simulink model "Simulink_Control_BlueROVtest6"  (R2022b)
settings: Solver=VariableStepAuto  StartTime=0.0  StopTime=20  RelTol=1e-3
model workspace (MAT data in the model file):
  Minv : Simulink.Parameter (value not decoded)
values from neighbouring files (symbols this model uses):
  B = 0    [Control_BlueROV_Modo_Deslizante.m]
  C = 1    [Control_BlueROV_Modo_Deslizante.m]
  epsilong = 1    [Control_BlueROV_Modo_Deslizante.m]
  Ix = 0.1836    [Control_BlueROV_Modo_Deslizante.m]
  Ixy = 0    [Control_BlueROV_Modo_Deslizante.m]
  Ixz = 0    [Control_BlueROV_Modo_Deslizante.m]
  Iy = 0.2181    [Control_BlueROV_Modo_Deslizante.m]
  Iyz = -0.0021    [Control_BlueROV_Modo_Deslizante.m]
  Iz = 0.1482    [Control_BlueROV_Modo_Deslizante.m]
  K = 5    [Control_BlueROV_Modo_Deslizante.m]
  Kp = -5.005    [Control_BlueROV_Modo_Deslizante.m]
  Kpdot = -0.8576    [Control_BlueROV_Modo_Deslizante.m]
  Kpp = -80.25    [Control_BlueROV_Modo_Deslizante.m]
  m = 10.7668    [Control_BlueROV_Modo_Deslizante.m]
  M = Mrb+Ma    [Control_BlueROV_Modo_Deslizante.m]
  Minv = inv(M)    [Control_BlueROV_Modo_Deslizante.m]
  Mq = -5.005    [Control_BlueROV_Modo_Deslizante.m]
  Mqdot = -1.1214    [Control_BlueROV_Modo_Deslizante.m]
  Mqq = -80.25    [Control_BlueROV_Modo_Deslizante.m]
  Nr = -0.004    [Control_BlueROV_Modo_Deslizante.m]
  Nrdot = -0.7399    [Control_BlueROV_Modo_Deslizante.m]
  Nrr = -0.2506    [Control_BlueROV_Modo_Deslizante.m]
  W = 0    [Control_BlueROV_Modo_Deslizante.m]
  xb = 0    [Control_BlueROV_Modo_Deslizante.m]
  xg = 0    [Control_BlueROV_Modo_Deslizante.m]
  Xu = -0.0048    [Control_BlueROV_Modo_Deslizante.m]
  Xudot = -4.9063    [Control_BlueROV_Modo_Deslizante.m]
  Xuu = -30.61    [Control_BlueROV_Modo_Deslizante.m]
  yb = 0    [Control_BlueROV_Modo_Deslizante.m]
  yg = 0    [Control_BlueROV_Modo_Deslizante.m]
  Yv = -0.2437    [Control_BlueROV_Modo_Deslizante.m]
  Yvdot = -9.9210    (= -9.921)    [Control_BlueROV_Modo_Deslizante.m]
  Yvv = -38.0036    [Control_BlueROV_Modo_Deslizante.m]
  zb = 0.02    [Control_BlueROV_Modo_Deslizante.m]
  zg = 0    [Control_BlueROV_Modo_Deslizante.m]
  Zw = -0.0094    [Control_BlueROV_Modo_Deslizante.m]
  Zwdot = -17.6159    [Control_BlueROV_Modo_Deslizante.m]
  Zww = -62.5364    [Control_BlueROV_Modo_Deslizante.m]
libraries: simulink x1
(part 2 of 3)

== system Simulink_Control_BlueROVtest6/BlueRov2Heavy/C(v)/Subsystem13 ==
  In1 : Inport
  In2 : Inport  Port=2
  In3 : Inport  Port=3
  In4 : Inport  Port=4
  Add4 : Sum  Inputs=+++
  Add8 : Sum
  Constant : Constant  Value=Iyz
  Constant1 : Constant  Value=-Iy
  Constant10 : Constant  Value=Ixy
  Constant11 : Constant  Value=Mqdot
  Product{1,19..21} (4 alike) : Product
  Out1 : Outport  VectorParamsAs1DForOutWhenUnconnected=off
  wires:
  In3/1 -> Product1/2
  In4/1 -> Product21/2
  Constant1/1 -> Product1/1
  Product1/1 -> Add4/3
  Product20/1 -> Add4/2
  Constant11/1 -> Product21/1
  Add4/1 -> Add8/1
  Product19/1 -> Add4/1
  Constant/1 -> Product19/1
  Product21/1 -> Add8/2
  Constant10/1 -> Product20/1
  Add8/1 -> Out1/1
  In1/1 -> Product19/2
  In2/1 -> Product20/2

== system Simulink_Control_BlueROVtest6/BlueRov2Heavy/C(v)/Subsystem14 ==
  In1 : Inport
  In2 : Inport  Port=2
  In3 : Inport  Port=3
  Add4 : Sum  Inputs=+-
  Add8 : Sum
  Constant : Constant  Value=xg
  Constant10 : Constant
  Constant11 : Constant  Value=Zwdot
  Gain : Gain  Gain=m
  Product19 : Product
  Product20 : Product
  Product21 : Product
  Out1 : Outport  VectorParamsAs1DForOutWhenUnconnected=off
  wires:
  Product20/1 -> Add4/2
  Constant11/1 -> Product21/1
  Gain/1 -> Add8/1
  Product19/1 -> Add4/1
  Constant/1 -> Product19/1
  Product21/1 -> Add8/2
  Add4/1 -> Gain/1
  Constant10/1 -> Product20/1
  Add8/1 -> Out1/1
  In1/1 -> Product19/2
  In3/1 -> Product21/2
  In2/1 -> Product20/2

== system Simulink_Control_BlueROVtest6/BlueRov2Heavy/C(v)/Subsystem15 ==
  In1 : Inport
  In2 : Inport  Port=2
  In3 : Inport  Port=3
  Add4 : Sum
  Add8 : Sum
  Constant : Constant  Value=zg
  Constant10 : Constant
  Constant11 : Constant  Value=-Xudot
  Gain : Gain  Gain=m
  Product19 : Product
  Product20 : Product
  Product21 : Product
  Out1 : Outport  VectorParamsAs1DForOutWhenUnconnected=off
  wires:
  In2/1 -> Product20/2
  In3/1 -> Product21/2
  In1/1 -> Product19/2
  Add8/1 -> Out1/1
  Constant10/1 -> Product20/1
  Add4/1 -> Gain/1
  Product21/1 -> Add8/2
  Constant/1 -> Product19/1
  Product19/1 -> Add4/1
  Gain/1 -> Add8/1
  Constant11/1 -> Product21/1
  Product20/1 -> Add4/2

== system Simulink_Control_BlueROVtest6/BlueRov2Heavy/C(v)/Subsystem16 ==
  In1 : Inport
  In2 : Inport  Port=2
  Add4 : Sum
  Constant : Constant  Value=zg
  Constant10 : Constant  Value=xg
  Gain : Gain  Gain=-m
  Product19 : Product
  Product20 : Product
  Out1 : Outport  VectorParamsAs1DForOutWhenUnconnected=off
  wires:
  Product20/1 -> Add4/2
  Product19/1 -> Add4/1
  In1/1 -> Product19/2
  Constant/1 -> Product19/1
  Gain/1 -> Out1/1
  Constant10/1 -> Product20/1
  Add4/1 -> Gain/1
  In2/1 -> Product20/2

== system Simulink_Control_BlueROVtest6/BlueRov2Heavy/C(v)/Subsystem17 ==
  In1 : Inport
  In2 : Inport  Port=2
  In3 : Inport  Port=3
  In4 : Inport  Port=4
  Add4 : Sum  Inputs=+++
  Add8 : Sum
  Constant : Constant  Value=Iyz
  Constant1 : Constant  Value=-Iz
  Constant10 : Constant  Value=Ixz
  Constant11 : Constant  Value=Nrdot
  Product{1,19..21} (4 alike) : Product
  Out1 : Outport  VectorParamsAs1DForOutWhenUnconnected=off
  wires:
  In3/1 -> Product1/2
  In4/1 -> Product21/2
  Constant1/1 -> Product1/1
  Product1/1 -> Add4/3
  Product20/1 -> Add4/2
  Constant11/1 -> Product21/1
  Add4/1 -> Add8/1
  Product19/1 -> Add4/1
  Constant/1 -> Product19/1
  Product21/1 -> Add8/2
  Constant10/1 -> Product20/1
  Add8/1 -> Out1/1
  In1/1 -> Product19/2
  In2/1 -> Product20/2

== system Simulink_Control_BlueROVtest6/BlueRov2Heavy/C(v)/Subsystem18 ==
  In1 : Inport
  In2 : Inport  Port=2
  In3 : Inport  Port=3
  In4 : Inport  Port=4
  Add4 : Sum  Inputs=+++
  Add8 : Sum
  Constant : Constant  Value=-Ixz
  Constant1 : Constant  Value=Ix
  Constant10 : Constant  Value=-Ixy
  Constant11 : Constant  Value=-Kpdot
  Product{1,19..21} (4 alike) : Product
  Out1 : Outport  VectorParamsAs1DForOutWhenUnconnected=off
  wires:
  In2/1 -> Product20/2
  In1/1 -> Product19/2
  Add8/1 -> Out1/1
  Constant10/1 -> Product20/1
  Product21/1 -> Add8/2
  Constant/1 -> Product19/1
  Product19/1 -> Add4/1
  Add4/1 -> Add8/1
  Constant11/1 -> Product21/1
  Product20/1 -> Add4/2
  Product1/1 -> Add4/3
  Constant1/1 -> Product1/1
  In4/1 -> Product21/2
  In3/1 -> Product1/2

== system Simulink_Control_BlueROVtest6/BlueRov2Heavy/C(v)/Subsystem19 ==
  In1 : Inport
  In2 : Inport  Port=2
  In3 : Inport  Port=3
  Add4 : Sum
  Add8 : Sum
  Constant : Constant  Value=xg
  Constant10 : Constant
  Constant11 : Constant  Value=-Yvdot
  Gain : Gain  Gain=m
  Product19 : Product
  Product20 : Product
  Product21 : Product
  Out1 : Outport  VectorParamsAs1DForOutWhenUnconnected=off
  wires:
  In2/1 -> Product20/2
  In3/1 -> Product21/2
  In1/1 -> Product19/2
  Add8/1 -> Out1/1
  Constant10/1 -> Product20/1
  Add4/1 -> Gain/1
  Product21/1 -> Add8/2
  Constant/1 -> Product19/1
  Product19/1 -> Add4/1
  Gain/1 -> Add8/1
  Constant11/1 -> Product21/1
  Product20/1 -> Add4/2

== system Simulink_Control_BlueROVtest6/BlueRov2Heavy/C(v)/Subsystem2 ==
  In1 : Inport
  In2 : Inport  Port=2
  In3 : Inport  Port=3
  Add10 : Sum  Inputs=-+
  Add9 : Sum
  Constant12 : Constant  Value=xg
  Constant13 : Constant
  Constant14 : Constant  Value=Yvdot
  Gain1 : Gain  Gain=m
  Product22 : Product
  Product23 : Product
  Product24 : Product
  Out1 : Outport  VectorParamsAs1DForOutWhenUnconnected=off
  wires:
  In1/1 -> Product22/2
  Constant14/1 -> Product24/1
  Add9/1 -> Gain1/1
  Constant12/1 -> Product22/1
  Product23/1 -> Add9/2
  Gain1/1 -> Add10/1
  Constant13/1 -> Product23/1
  Product24/1 -> Add10/2
  Product22/1 -> Add9/1
  In3/1 -> Product24/2
  Add10/1 -> Out1/1
  In2/1 -> Product23/2

== system Simulink_Control_BlueROVtest6/BlueRov2Heavy/C(v)/Subsystem20 ==
  In1 : Inport
  In2 : Inport  Port=2
  In3 : Inport  Port=3
  Add4 : Sum
  Add8 : Sum
  Constant : Constant  Value=yg
  Constant10 : Constant  Value=-1
  Constant11 : Constant  Value=Xudot
  Gain : Gain  Gain=m
  Product19 : Product
  Product20 : Product
  Product21 : Product
  Out1 : Outport  VectorParamsAs1DForOutWhenUnconnected=off
  wires:
  Product20/1 -> Add4/2
  Constant11/1 -> Product21/1
  Gain/1 -> Add8/1
  Product19/1 -> Add4/1
  Constant/1 -> Product19/1
  Product21/1 -> Add8/2
  Add4/1 -> Gain/1
  Constant10/1 -> Product20/1
  Add8/1 -> Out1/1
  In1/1 -> Product19/2
  In3/1 -> Product21/2
  In2/1 -> Product20/2

== system Simulink_Control_BlueROVtest6/BlueRov2Heavy/C(v)/Subsystem21 ==
  In1 : Inport
  In2 : Inport  Port=2
  Add4 : Sum
  Constant : Constant  Value=xg
  Constant10 : Constant  Value=yg
  Gain : Gain  Gain=-m
  Product19 : Product
  Product20 : Product
  Out1 : Outport  VectorParamsAs1DForOutWhenUnconnected=off
  wires:
  In2/1 -> Product20/2
  Add4/1 -> Gain/1
  Constant10/1 -> Product20/1
  Gain/1 -> Out1/1
  Constant/1 -> Product19/1
  In1/1 -> Product19/2
  Product19/1 -> Add4/1
  Product20/1 -> Add4/2

== system Simulink_Control_BlueROVtest6/BlueRov2Heavy/C(v)/Subsystem22 ==
  In1 : Inport
  In2 : Inport  Port=2
  In3 : Inport  Port=3
  In4 : Inport  Port=4
  Add4 : Sum  Inputs=+++
  Add8 : Sum
  Constant : Constant  Value=-Iyz
  Constant1 : Constant  Value=Iy
  Constant10 : Constant  Value=-Ixy
  Constant11 : Constant  Value=-Mqdot
  Product{1,19..21} (4 alike) : Product
  Out1 : Outport  VectorParamsAs1DForOutWhenUnconnected=off
  wires:
  In2/1 -> Product20/2
  In1/1 -> Product19/2
  Add8/1 -> Out1/1
  Constant10/1 -> Product20/1
  Product21/1 -> Add8/2
  Constant/1 -> Product19/1
  Product19/1 -> Add4/1
  Add4/1 -> Add8/1
  Constant11/1 -> Product21/1
  Product20/1 -> Add4/2
  Product1/1 -> Add4/3
  Constant1/1 -> Product1/1
  In4/1 -> Product21/2
  In3/1 -> Product1/2

== system Simulink_Control_BlueROVtest6/BlueRov2Heavy/C(v)/Subsystem23 ==
  In1 : Inport
  In2 : Inport  Port=2
  In3 : Inport  Port=3
  In4 : Inport  Port=4
  Add4 : Sum  Inputs=+++
  Add8 : Sum
  Constant : Constant  Value=Ixz
  Constant1 : Constant  Value=-Ix
  Constant10 : Constant  Value=Ixy
  Constant11 : Constant  Value=Kpdot
  Product{1,19..21} (4 alike) : Product
  Out1 : Outport  VectorParamsAs1DForOutWhenUnconnected=off
  wires:
  In3/1 -> Product1/2
  In4/1 -> Product21/2
  Constant1/1 -> Product1/1
  Product1/1 -> Add4/3
  Product20/1 -> Add4/2
  Constant11/1 -> Product21/1
  Add4/1 -> Add8/1
  Product19/1 -> Add4/1
  Constant/1 -> Product19/1
  Product21/1 -> Add8/2
  Constant10/1 -> Product20/1
  Add8/1 -> Out1/1
  In1/1 -> Product19/2
  In2/1 -> Product20/2

== system Simulink_Control_BlueROVtest6/BlueRov2Heavy/C(v)/Subsystem3 ==
  In1 : Inport
  In2 : Inport  Port=2
  In3 : Inport  Port=3
  Add4 : Sum
  Add8 : Sum  Inputs=-+
  Constant : Constant  Value=yg
  Constant10 : Constant
  Constant11 : Constant  Value=Zwdot
  Gain : Gain  Gain=m
  Product19 : Product
  Product20 : Product
  Product21 : Product
  Out1 : Outport  VectorParamsAs1DForOutWhenUnconnected=off
  wires:
  In2/1 -> Product20/2
  In3/1 -> Product21/2
  In1/1 -> Product19/2
  Add8/1 -> Out1/1
  Constant10/1 -> Product20/1
  Add4/1 -> Gain/1
  Product21/1 -> Add8/2
  Constant/1 -> Product19/1
  Product19/1 -> Add4/1
  Gain/1 -> Add8/1
  Constant11/1 -> Product21/1
  Product20/1 -> Add4/2

== system Simulink_Control_BlueROVtest6/BlueRov2Heavy/C(v)/Subsystem4 ==
  In1 : Inport
  In2 : Inport  Port=2
  Add4 : Sum
  Constant : Constant  Value=zg
  Constant10 : Constant  Value=xg
  Gain : Gain  Gain=m
  Product19 : Product
  Product20 : Product
  Out1 : Outport  VectorParamsAs1DForOutWhenUnconnected=off
  wires:
  In2/1 -> Product20/2
  Add4/1 -> Gain/1
  Constant10/1 -> Product20/1
  Gain/1 -> Out1/1
  Constant/1 -> Product19/1
  In1/1 -> Product19/2
  Product19/1 -> Add4/1
  Product20/1 -> Add4/2

== system Simulink_Control_BlueROVtest6/BlueRov2Heavy/C(v)/Subsystem5 ==
  In1 : Inport
  In2 : Inport  Port=2
  In3 : Inport  Port=3
  Add4 : Sum  Inputs=+-
  Add8 : Sum  Inputs=-+
  Constant : Constant  Value=yg
  Constant10 : Constant
  Constant11 : Constant  Value=-Xudot
  Gain : Gain  Gain=m
  Product19 : Product
  Product20 : Product
  Product21 : Product
  Out1 : Outport  VectorParamsAs1DForOutWhenUnconnected=off
  wires:
  Product20/1 -> Add4/2
  Constant11/1 -> Product21/1
  Gain/1 -> Add8/1
  Product19/1 -> Add4/1
  Constant/1 -> Product19/1
  Product21/1 -> Add8/2
  Add4/1 -> Gain/1
  Constant10/1 -> Product20/1
  Add8/1 -> Out1/1
  In1/1 -> Product19/2
  In3/1 -> Product21/2
  In2/1 -> Product20/2

== system Simulink_Control_BlueROVtest6/BlueRov2Heavy/C(v)/Subsystem6 ==
  In1 : Inport
  In2 : Inport  Port=2
  In3 : Inport  Port=3
  Add4 : Sum  Inputs=+-
  Add8 : Sum  Inputs=-+
  Constant : Constant  Value=zg
  Constant10 : Constant
  Constant11 : Constant  Value=-Yvdot
  Gain : Gain  Gain=m
  Product19 : Product
  Product20 : Product
  Product21 : Product
  Out1 : Outport  VectorParamsAs1DForOutWhenUnconnected=off
  wires:
  In2/1 -> Product20/2
  In3/1 -> Product21/2
  In1/1 -> Product19/2
  Add8/1 -> Out1/1
  Constant10/1 -> Product20/1
  Add4/1 -> Gain/1
  Product21/1 -> Add8/2
  Constant/1 -> Product19/1
  Product19/1 -> Add4/1
  Gain/1 -> Add8/1
  Constant11/1 -> Product21/1
  Product20/1 -> Add4/2

== system Simulink_Control_BlueROVtest6/BlueRov2Heavy/C(v)/Subsystem7 ==
  In1 : Inport
  In2 : Inport  Port=2
  In3 : Inport  Port=3
  Add4 : Sum
  Add8 : Sum  Inputs=-+
  Constant : Constant  Value=zg
  Constant10 : Constant
  Constant11 : Constant  Value=Xudot
  Gain : Gain  Gain=m
  Product19 : Product
  Product20 : Product
  Product21 : Product
  Out1 : Outport  VectorParamsAs1DForOutWhenUnconnected=off
  wires:
  Product20/1 -> Add4/2
  Constant11/1 -> Product21/1
  Gain/1 -> Add8/1
  Product19/1 -> Add4/1
  Constant/1 -> Product19/1
  Product21/1 -> Add8/2
  Add4/1 -> Gain/1
  Constant10/1 -> Product20/1
  Add8/1 -> Out1/1
  In1/1 -> Product19/2
  In3/1 -> Product21/2
  In2/1 -> Product20/2

== system Simulink_Control_BlueROVtest6/BlueRov2Heavy/C(v)/Subsystem8 ==
  In1 : Inport
  In2 : Inport  Port=2
  Add4 : Sum
  Constant : Constant  Value=xg
  Constant10 : Constant  Value=yg
  Gain : Gain  Gain=m
  Product19 : Product
  Product20 : Product
  Out1 : Outport  VectorParamsAs1DForOutWhenUnconnected=off
  wires:
  In2/1 -> Product20/2
  Add4/1 -> Gain/1
  Constant10/1 -> Product20/1
  Gain/1 -> Out1/1
  Constant/1 -> Product19/1
  In1/1 -> Product19/2
  Product19/1 -> Add4/1
  Product20/1 -> Add4/2

== system Simulink_Control_BlueROVtest6/BlueRov2Heavy/C(v)/Subsystem9 ==
  In1 : Inport
  In2 : Inport  Port=2
  Add4 : Sum
  Constant : Constant  Value=yg
  Constant10 : Constant  Value=zg
  Gain : Gain  Gain=-m
  Product19 : Product
  Product20 : Product
  Out1 : Outport  VectorParamsAs1DForOutWhenUnconnected=off
  wires:
  In2/1 -> Product20/2
  Add4/1 -> Gain/1
  Constant10/1 -> Product20/1
  Gain/1 -> Out1/1
  Constant/1 -> Product19/1
  In1/1 -> Product19/2
  Product19/1 -> Add4/1
  Product20/1 -> Add4/2

== system Simulink_Control_BlueROVtest6/BlueRov2Heavy/J(n)/Subsystem1 ==
  In1 : Inport
  In2 : Inport  Port=2
  Product6 : Product
  Out1 : Outport  VectorParamsAs1DForOutWhenUnconnected=off
  wires:
  In1/1 -> Product6/1
  In2/1 -> Product6/2
  Product6/1 -> Out1/1

== system Simulink_Control_BlueROVtest6/BlueRov2Heavy/J(n)/Subsystem10 ==
  In1 : Inport
  In2 : Inport  Port=2
  Product6 : Product
  Out1 : Outport  VectorParamsAs1DForOutWhenUnconnected=off
  wires:
  In1/1 -> Product6/1
  In2/1 -> Product6/2
  Product6/1 -> Out1/1

== system Simulink_Control_BlueROVtest6/BlueRov2Heavy/J(n)/Subsystem11 ==
  In1 : Inport
  In2 : Inport  Port=2
  Product6 : Product
  Out1 : Outport  VectorParamsAs1DForOutWhenUnconnected=off
  wires:
  In1/1 -> Product6/1
  In2/1 -> Product6/2
  Product6/1 -> Out1/1

== system Simulink_Control_BlueROVtest6/BlueRov2Heavy/J(n)/Subsystem12 ==
  In1 : Inport
  In2 : Inport  Port=2
  Product6 : Product
  Out1 : Outport  VectorParamsAs1DForOutWhenUnconnected=off
  wires:
  In1/1 -> Product6/1
  In2/1 -> Product6/2
  Product6/1 -> Out1/1

== system Simulink_Control_BlueROVtest6/BlueRov2Heavy/J(n)/Subsystem2 ==
  In1 : Inport
  In2 : Inport  Port=2
  In3 : Inport  Port=3
  In4 : Inport  Port=4
  In5 : Inport  Port=5
  Add7 : Sum
  Product37 : Product
  Product38 : Product  Inputs=3
  Out1 : Outport  VectorParamsAs1DForOutWhenUnconnected=off
  wires:
  In5/1 -> Product38/3
  In4/1 -> Product38/2
  In3/1 -> Product38/1
  In2/1 -> Product37/2
  In1/1 -> Product37/1
  Product37/1 -> Add7/1
  Add7/1 -> Out1/1
  Product38/1 -> Add7/2

== system Simulink_Control_BlueROVtest6/BlueRov2Heavy/J(n)/Subsystem3 ==
  In1 : Inport
  In2 : Inport  Port=2
  Product6 : Product
  Out1 : Outport  VectorParamsAs1DForOutWhenUnconnected=off
  wires:
  Product6/1 -> Out1/1
  In2/1 -> Product6/2
  In1/1 -> Product6/1

== system Simulink_Control_BlueROVtest6/BlueRov2Heavy/J(n)/Subsystem4 ==
  In1 : Inport
  In2 : Inport  Port=2
  In3 : Inport  Port=3
  In4 : Inport  Port=4
  In5 : Inport  Port=5
  Add7 : Sum  Inputs=-+
  Product37 : Product
  Product38 : Product  Inputs=3
  Out1 : Outport  VectorParamsAs1DForOutWhenUnconnected=off
  wires:
  Product38/1 -> Add7/2
  Add7/1 -> Out1/1
  Product37/1 -> Add7/1
  In1/1 -> Product37/1
  In2/1 -> Product37/2
  In3/1 -> Product38/1
  In4/1 -> Product38/2
  In5/1 -> Product38/3

== system Simulink_Control_BlueROVtest6/BlueRov2Heavy/J(n)/Subsystem5 ==
  In1 : Inport
  In2 : Inport  Port=2
  In3 : Inport  Port=3
  In4 : Inport  Port=4
  In5 : Inport  Port=5
  Add7 : Sum
  Product37 : Product
  Product38 : Product  Inputs=3
  Out1 : Outport  VectorParamsAs1DForOutWhenUnconnected=off
  wires:
  Product38/1 -> Add7/2
  Add7/1 -> Out1/1
  Product37/1 -> Add7/1
  In1/1 -> Product37/1
  In2/1 -> Product37/2
  In3/1 -> Product38/1
  In4/1 -> Product38/2
  In5/1 -> Product38/3

== system Simulink_Control_BlueROVtest6/BlueRov2Heavy/J(n)/Subsystem6 ==
  In1 : Inport
  In2 : Inport  Port=2
  In3 : Inport  Port=3
  In4 : Inport  Port=4
  In5 : Inport  Port=5
  Add7 : Sum  Inputs=-+
  Product37 : Product
  Product38 : Product  Inputs=3
  Out1 : Outport  VectorParamsAs1DForOutWhenUnconnected=off
  wires:
  In5/1 -> Product38/3
  In4/1 -> Product38/2
  In3/1 -> Product38/1
  In2/1 -> Product37/2
  In1/1 -> Product37/1
  Product37/1 -> Add7/1
  Add7/1 -> Out1/1
  Product38/1 -> Add7/2

== system Simulink_Control_BlueROVtest6/BlueRov2Heavy/J(n)/Subsystem7 ==
  In1 : Inport
  In2 : Inport  Port=2
  Product6 : Product
  Out1 : Outport  VectorParamsAs1DForOutWhenUnconnected=off
  wires:
  In1/1 -> Product6/1
  In2/1 -> Product6/2
  Product6/1 -> Out1/1

== system Simulink_Control_BlueROVtest6/BlueRov2Heavy/J(n)/Subsystem8 ==
  In1 : Inport
  In2 : Inport  Port=2
  Product6 : Product
  Out1 : Outport  VectorParamsAs1DForOutWhenUnconnected=off
  wires:
  Product6/1 -> Out1/1
  In2/1 -> Product6/2
  In1/1 -> Product6/1

== system Simulink_Control_BlueROVtest6/BlueRov2Heavy/J(n)/Subsystem9 ==
  In1 : Inport
  In2 : Inport  Port=2
  Product6 : Product
  Out1 : Outport  VectorParamsAs1DForOutWhenUnconnected=off
  wires:
  In1/1 -> Product6/1
  In2/1 -> Product6/2
  Product6/1 -> Out1/1

== system Simulink_Control_BlueROVtest6/FeedBackData1/J(n)/Subsystem1 ==
  In1 : Inport
  In2 : Inport  Port=2
  Product6 : Product
  Out1 : Outport  VectorParamsAs1DForOutWhenUnconnected=off
  wires:
  In1/1 -> Product6/1
  In2/1 -> Product6/2
  Product6/1 -> Out1/1

== system Simulink_Control_BlueROVtest6/FeedBackData1/J(n)/Subsystem10 ==
  In1 : Inport
  In2 : Inport  Port=2
  Product6 : Product
  Out1 : Outport  VectorParamsAs1DForOutWhenUnconnected=off
  wires:
  In1/1 -> Product6/1
  In2/1 -> Product6/2
  Product6/1 -> Out1/1

== system Simulink_Control_BlueROVtest6/FeedBackData1/J(n)/Subsystem11 ==
  In1 : Inport
  In2 : Inport  Port=2
  Product6 : Product
  Out1 : Outport  VectorParamsAs1DForOutWhenUnconnected=off
  wires:
  In1/1 -> Product6/1
  In2/1 -> Product6/2
  Product6/1 -> Out1/1

== system Simulink_Control_BlueROVtest6/FeedBackData1/J(n)/Subsystem12 ==
  In1 : Inport
  In2 : Inport  Port=2
  Product6 : Product
  Out1 : Outport  VectorParamsAs1DForOutWhenUnconnected=off
  wires:
  In1/1 -> Product6/1
  In2/1 -> Product6/2
  Product6/1 -> Out1/1

== system Simulink_Control_BlueROVtest6/FeedBackData1/J(n)/Subsystem2 ==
  In1 : Inport
  In2 : Inport  Port=2
  In3 : Inport  Port=3
  In4 : Inport  Port=4
  In5 : Inport  Port=5
  Add7 : Sum
  Product37 : Product
  Product38 : Product  Inputs=3
  Out1 : Outport  VectorParamsAs1DForOutWhenUnconnected=off
  wires:
  In5/1 -> Product38/3
  In4/1 -> Product38/2
  In3/1 -> Product38/1
  In2/1 -> Product37/2
  In1/1 -> Product37/1
  Product37/1 -> Add7/1
  Add7/1 -> Out1/1
  Product38/1 -> Add7/2

== system Simulink_Control_BlueROVtest6/FeedBackData1/J(n)/Subsystem3 ==
  In1 : Inport
  In2 : Inport  Port=2
  Product6 : Product
  Out1 : Outport  VectorParamsAs1DForOutWhenUnconnected=off
  wires:
  Product6/1 -> Out1/1
  In2/1 -> Product6/2
  In1/1 -> Product6/1

== system Simulink_Control_BlueROVtest6/FeedBackData1/J(n)/Subsystem4 ==
  In1 : Inport
  In2 : Inport  Port=2
  In3 : Inport  Port=3
  In4 : Inport  Port=4
  In5 : Inport  Port=5
  Add7 : Sum  Inputs=-+
  Product37 : Product
  Product38 : Product  Inputs=3
  Out1 : Outport  VectorParamsAs1DForOutWhenUnconnected=off
  wires:
  Product38/1 -> Add7/2
  Add7/1 -> Out1/1
  Product37/1 -> Add7/1
  In1/1 -> Product37/1
  In2/1 -> Product37/2
  In3/1 -> Product38/1
  In4/1 -> Product38/2
  In5/1 -> Product38/3

== system Simulink_Control_BlueROVtest6/FeedBackData1/J(n)/Subsystem5 ==
  In1 : Inport
  In2 : Inport  Port=2
  In3 : Inport  Port=3
  In4 : Inport  Port=4
  In5 : Inport  Port=5
  Add7 : Sum
  Product37 : Product
  Product38 : Product  Inputs=3
  Out1 : Outport  VectorParamsAs1DForOutWhenUnconnected=off
  wires:
  Product38/1 -> Add7/2
  Add7/1 -> Out1/1
  Product37/1 -> Add7/1
  In1/1 -> Product37/1
  In2/1 -> Product37/2
  In3/1 -> Product38/1
  In4/1 -> Product38/2
  In5/1 -> Product38/3

== system Simulink_Control_BlueROVtest6/FeedBackData1/J(n)/Subsystem6 ==
  In1 : Inport
  In2 : Inport  Port=2
  In3 : Inport  Port=3
  In4 : Inport  Port=4
  In5 : Inport  Port=5
  Add7 : Sum  Inputs=-+
  Product37 : Product
  Product38 : Product  Inputs=3
  Out1 : Outport  VectorParamsAs1DForOutWhenUnconnected=off
  wires:
  In5/1 -> Product38/3
  In4/1 -> Product38/2
  In3/1 -> Product38/1
  In2/1 -> Product37/2
  In1/1 -> Product37/1
  Product37/1 -> Add7/1
  Add7/1 -> Out1/1
  Product38/1 -> Add7/2

== system Simulink_Control_BlueROVtest6/FeedBackData1/J(n)/Subsystem7 ==
  In1 : Inport
  In2 : Inport  Port=2
  Product6 : Product
  Out1 : Outport  VectorParamsAs1DForOutWhenUnconnected=off
  wires:
  In1/1 -> Product6/1
  In2/1 -> Product6/2
  Product6/1 -> Out1/1

== system Simulink_Control_BlueROVtest6/FeedBackData1/J(n)/Subsystem8 ==
  In1 : Inport
  In2 : Inport  Port=2
  Product6 : Product
  Out1 : Outport  VectorParamsAs1DForOutWhenUnconnected=off
  wires:
  Product6/1 -> Out1/1
  In2/1 -> Product6/2
  In1/1 -> Product6/1

== system Simulink_Control_BlueROVtest6/FeedBackData1/J(n)/Subsystem9 ==
  In1 : Inport
  In2 : Inport  Port=2
  Product6 : Product
  Out1 : Outport  VectorParamsAs1DForOutWhenUnconnected=off
  wires:
  In1/1 -> Product6/1
  In2/1 -> Product6/2
  Product6/1 -> Out1/1

== system Simulink_Control_BlueROVtest6/Sliding Mode Control/C(v)/Subsystem ==
  In1 : Inport
  In2 : Inport  Port=2
  Add4 : Sum
  Constant : Constant  Value=zg
  Constant10 : Constant  Value=yg
  Gain : Gain  Gain=m
  Product19 : Product
  Product20 : Product
  Out1 : Outport  VectorParamsAs1DForOutWhenUnconnected=off
  wires:
  Product20/1 -> Add4/2
  Product19/1 -> Add4/1
  In1/1 -> Product19/2
  Constant/1 -> Product19/1
  Gain/1 -> Out1/1
  Constant10/1 -> Product20/1
  Add4/1 -> Gain/1
  In2/1 -> Product20/2

== system Simulink_Control_BlueROVtest6/Sliding Mode Control/C(v)/Subsystem1 ==
  In1 : Inport
  In2 : Inport  Port=2
  In3 : Inport  Port=3
  Add4 : Sum  Inputs=+-
  Add8 : Sum  Inputs=-+
  Constant : Constant  Value=xg
  Constant10 : Constant
  Constant11 : Constant  Value=-Zwdot
  Gain : Gain  Gain=m
  Product19 : Product
  Product20 : Product
  Product21 : Product
  Out1 : Outport  VectorParamsAs1DForOutWhenUnconnected=off
  wires:
  Product20/1 -> Add4/2
  Constant11/1 -> Product21/1
  Gain/1 -> Add8/1
  Product19/1 -> Add4/1
  Constant/1 -> Product19/1
  Product21/1 -> Add8/2
  Add4/1 -> Gain/1
  Constant10/1 -> Product20/1
  Add8/1 -> Out1/1
  In1/1 -> Product19/2
  In3/1 -> Product21/2
  In2/1 -> Product20/2

== system Simulink_Control_BlueROVtest6/Sliding Mode Control/C(v)/Subsystem10 ==
  In1 : Inport
  In2 : Inport  Port=2
  In3 : Inport  Port=3
  Add4 : Sum
  Add8 : Sum
  Constant : Constant  Value=yg
  Constant10 : Constant
  Constant11 : Constant  Value=-Zwdot
  Gain : Gain  Gain=m
  Product19 : Product
  Product20 : Product
  Product21 : Product
  Out1 : Outport  VectorParamsAs1DForOutWhenUnconnected=off
  wires:
  In2/1 -> Product20/2
  In3/1 -> Product21/2
  In1/1 -> Product19/2
  Add8/1 -> Out1/1
  Constant10/1 -> Product20/1
  Add4/1 -> Gain/1
  Product21/1 -> Add8/2
  Constant/1 -> Product19/1
  Product19/1 -> Add4/1
  Gain/1 -> Add8/1
  Constant11/1 -> Product21/1
  Product20/1 -> Add4/2

== system Simulink_Control_BlueROVtest6/Sliding Mode Control/C(v)/Subsystem11 ==
  In1 : Inport
  In2 : Inport  Port=2
  In3 : Inport  Port=3
  Add4 : Sum  Inputs=+-
  Add8 : Sum
  Constant : Constant  Value=zg
  Constant10 : Constant
  Constant11 : Constant  Value=Yvdot
  Gain : Gain  Gain=m
  Product19 : Product
  Product20 : Product
  Product21 : Product
  Out1 : Outport  VectorParamsAs1DForOutWhenUnconnected=off
  wires:
  Product20/1 -> Add4/2
  Constant11/1 -> Product21/1
  Gain/1 -> Add8/1
  Product19/1 -> Add4/1
  Constant/1 -> Product19/1
  Product21/1 -> Add8/2
  Add4/1 -> Gain/1
  Constant10/1 -> Product20/1
  Add8/1 -> Out1/1
  In1/1 -> Product19/2
  In3/1 -> Product21/2
  In2/1 -> Product20/2

== system Simulink_Control_BlueROVtest6/Sliding Mode Control/C(v)/Subsystem12 ==
  In1 : Inport
  In2 : Inport  Port=2
  In3 : Inport  Port=3
  In4 : Inport  Port=4
  Add4 : Sum  Inputs=+++
  Add8 : Sum
  Constant : Constant  Value=-Iyz
  Constant1 : Constant  Value=Iz
  Constant10 : Constant  Value=-Ixz
  Constant11 : Constant  Value=-Nrdot
  Product{1,19..21} (4 alike) : Product
  Out1 : Outport  VectorParamsAs1DForOutWhenUnconnected=off
  wires:
  In2/1 -> Product20/2
  In1/1 -> Product19/2
  Add8/1 -> Out1/1
  Constant10/1 -> Product20/1
  Product21/1 -> Add8/2
  Constant/1 -> Product19/1
  Product19/1 -> Add4/1
  Add4/1 -> Add8/1
  Constant11/1 -> Product21/1
  Product20/1 -> Add4/2
  Product1/1 -> Add4/3
  Constant1/1 -> Product1/1
  In4/1 -> Product21/2
  In3/1 -> Product1/2

== system Simulink_Control_BlueROVtest6/Sliding Mode Control/C(v)/Subsystem13 ==
  In1 : Inport
  In2 : Inport  Port=2
  In3 : Inport  Port=3
  In4 : Inport  Port=4
  Add4 : Sum  Inputs=+++
  Add8 : Sum
  Constant : Constant  Value=Iyz
  Constant1 : Constant  Value=-Iy
  Constant10 : Constant  Value=Ixy
  Constant11 : Constant  Value=Mqdot
  Product{1,19..21} (4 alike) : Product
  Out1 : Outport  VectorParamsAs1DForOutWhenUnconnected=off
  wires:
  In3/1 -> Product1/2
  In4/1 -> Product21/2
  Constant1/1 -> Product1/1
  Product1/1 -> Add4/3
  Product20/1 -> Add4/2
  Constant11/1 -> Product21/1
  Add4/1 -> Add8/1
  Product19/1 -> Add4/1
  Constant/1 -> Product19/1
  Product21/1 -> Add8/2
  Constant10/1 -> Product20/1
  Add8/1 -> Out1/1
  In1/1 -> Product19/2
  In2/1 -> Product20/2

== system Simulink_Control_BlueROVtest6/Sliding Mode Control/C(v)/Subsystem14 ==
  In1 : Inport
  In2 : Inport  Port=2
  In3 : Inport  Port=3
  Add4 : Sum  Inputs=+-
  Add8 : Sum
  Constant : Constant  Value=xg
  Constant10 : Constant
  Constant11 : Constant  Value=Zwdot
  Gain : Gain  Gain=m
  Product19 : Product
  Product20 : Product
  Product21 : Product
  Out1 : Outport  VectorParamsAs1DForOutWhenUnconnected=off
  wires:
  Product20/1 -> Add4/2
  Constant11/1 -> Product21/1
  Gain/1 -> Add8/1
  Product19/1 -> Add4/1
  Constant/1 -> Product19/1
  Product21/1 -> Add8/2
  Add4/1 -> Gain/1
  Constant10/1 -> Product20/1
  Add8/1 -> Out1/1
  In1/1 -> Product19/2
  In3/1 -> Product21/2
  In2/1 -> Product20/2

== system Simulink_Control_BlueROVtest6/Sliding Mode Control/C(v)/Subsystem15 ==
  In1 : Inport
  In2 : Inport  Port=2
  In3 : Inport  Port=3
  Add4 : Sum
  Add8 : Sum
  Constant : Constant  Value=zg
  Constant10 : Constant
  Constant11 : Constant  Value=-Xudot
  Gain : Gain  Gain=m
  Product19 : Product
  Product20 : Product
  Product21 : Product
  Out1 : Outport  VectorParamsAs1DForOutWhenUnconnected=off
  wires:
  In2/1 -> Product20/2
  In3/1 -> Product21/2
  In1/1 -> Product19/2
  Add8/1 -> Out1/1
  Constant10/1 -> Product20/1
  Add4/1 -> Gain/1
  Product21/1 -> Add8/2
  Constant/1 -> Product19/1
  Product19/1 -> Add4/1
  Gain/1 -> Add8/1
  Constant11/1 -> Product21/1
  Product20/1 -> Add4/2

== system Simulink_Control_BlueROVtest6/Sliding Mode Control/C(v)/Subsystem16 ==
  In1 : Inport
  In2 : Inport  Port=2
  Add4 : Sum
  Constant : Constant  Value=zg
  Constant10 : Constant  Value=xg
  Gain : Gain  Gain=-m
  Product19 : Product
  Product20 : Product
  Out1 : Outport  VectorParamsAs1DForOutWhenUnconnected=off
  wires:
  Product20/1 -> Add4/2
  Product19/1 -> Add4/1
  In1/1 -> Product19/2
  Constant/1 -> Product19/1
  Gain/1 -> Out1/1
  Constant10/1 -> Product20/1
  Add4/1 -> Gain/1
  In2/1 -> Product20/2

== system Simulink_Control_BlueROVtest6/Sliding Mode Control/C(v)/Subsystem17 ==
  In1 : Inport
  In2 : Inport  Port=2
  In3 : Inport  Port=3
  In4 : Inport  Port=4
  Add4 : Sum  Inputs=+++
  Add8 : Sum
  Constant : Constant  Value=Iyz
  Constant1 : Constant  Value=-Iz
  Constant10 : Constant  Value=Ixz
  Constant11 : Constant  Value=Nrdot
  Product{1,19..21} (4 alike) : Product
  Out1 : Outport  VectorParamsAs1DForOutWhenUnconnected=off
  wires:
  In3/1 -> Product1/2
  In4/1 -> Product21/2
  Constant1/1 -> Product1/1
  Product1/1 -> Add4/3
  Product20/1 -> Add4/2
  Constant11/1 -> Product21/1
  Add4/1 -> Add8/1
  Product19/1 -> Add4/1
  Constant/1 -> Product19/1
  Product21/1 -> Add8/2
  Constant10/1 -> Product20/1
  Add8/1 -> Out1/1
  In1/1 -> Product19/2
  In2/1 -> Product20/2

== system Simulink_Control_BlueROVtest6/Sliding Mode Control/C(v)/Subsystem18 ==
  In1 : Inport
  In2 : Inport  Port=2
  In3 : Inport  Port=3
  In4 : Inport  Port=4
  Add4 : Sum  Inputs=+++
  Add8 : Sum
  Constant : Constant  Value=-Ixz
  Constant1 : Constant  Value=Ix
  Constant10 : Constant  Value=-Ixy
  Constant11 : Constant  Value=-Kpdot
  Product{1,19..21} (4 alike) : Product
  Out1 : Outport  VectorParamsAs1DForOutWhenUnconnected=off
  wires:
  In2/1 -> Product20/2
  In1/1 -> Product19/2
  Add8/1 -> Out1/1
  Constant10/1 -> Product20/1
  Product21/1 -> Add8/2
  Constant/1 -> Product19/1
  Product19/1 -> Add4/1
  Add4/1 -> Add8/1
  Constant11/1 -> Product21/1
  Product20/1 -> Add4/2
  Product1/1 -> Add4/3
  Constant1/1 -> Product1/1
  In4/1 -> Product21/2
  In3/1 -> Product1/2

== system Simulink_Control_BlueROVtest6/Sliding Mode Control/C(v)/Subsystem19 ==
  In1 : Inport
  In2 : Inport  Port=2
  In3 : Inport  Port=3
  Add4 : Sum
  Add8 : Sum
  Constant : Constant  Value=xg
  Constant10 : Constant
  Constant11 : Constant  Value=-Yvdot
  Gain : Gain  Gain=m
  Product19 : Product
  Product20 : Product
  Product21 : Product
  Out1 : Outport  VectorParamsAs1DForOutWhenUnconnected=off
  wires:
  In2/1 -> Product20/2
  In3/1 -> Product21/2
  In1/1 -> Product19/2
  Add8/1 -> Out1/1
  Constant10/1 -> Product20/1
  Add4/1 -> Gain/1
  Product21/1 -> Add8/2
  Constant/1 -> Product19/1
  Product19/1 -> Add4/1
  Gain/1 -> Add8/1
  Constant11/1 -> Product21/1
  Product20/1 -> Add4/2

== system Simulink_Control_BlueROVtest6/Sliding Mode Control/C(v)/Subsystem2 ==
  In1 : Inport
  In2 : Inport  Port=2
  In3 : Inport  Port=3
  Add10 : Sum  Inputs=-+
  Add9 : Sum
  Constant12 : Constant  Value=xg
  Constant13 : Constant
  Constant14 : Constant  Value=Yvdot
  Gain1 : Gain  Gain=m
  Product22 : Product
  Product23 : Product
  Product24 : Product
  Out1 : Outport  VectorParamsAs1DForOutWhenUnconnected=off
  wires:
  In1/1 -> Product22/2
  Constant14/1 -> Product24/1
  Add9/1 -> Gain1/1
  Constant12/1 -> Product22/1
  Product23/1 -> Add9/2
  Gain1/1 -> Add10/1
  Constant13/1 -> Product23/1
  Product24/1 -> Add10/2
  Product22/1 -> Add9/1
  In3/1 -> Product24/2
  Add10/1 -> Out1/1
  In2/1 -> Product23/2

== system Simulink_Control_BlueROVtest6/Sliding Mode Control/C(v)/Subsystem20 ==
  In1 : Inport
  In2 : Inport  Port=2
  In3 : Inport  Port=3
  Add4 : Sum
  Add8 : Sum
  Constant : Constant  Value=yg
  Constant10 : Constant  Value=-1
  Constant11 : Constant  Value=Xudot
  Gain : Gain  Gain=m
  Product19 : Product
  Product20 : Product
  Product21 : Product
  Out1 : Outport  VectorParamsAs1DForOutWhenUnconnected=off
  wires:
  Product20/1 -> Add4/2
  Constant11/1 -> Product21/1
  Gain/1 -> Add8/1
  Product19/1 -> Add4/1
  Constant/1 -> Product19/1
  Product21/1 -> Add8/2
  Add4/1 -> Gain/1
  Constant10/1 -> Product20/1
  Add8/1 -> Out1/1
  In1/1 -> Product19/2
  In3/1 -> Product21/2
  In2/1 -> Product20/2

== system Simulink_Control_BlueROVtest6/Sliding Mode Control/C(v)/Subsystem21 ==
  In1 : Inport
  In2 : Inport  Port=2
  Add4 : Sum
  Constant : Constant  Value=xg
  Constant10 : Constant  Value=yg
  Gain : Gain  Gain=-m
  Product19 : Product
  Product20 : Product
  Out1 : Outport  VectorParamsAs1DForOutWhenUnconnected=off
  wires:
  In2/1 -> Product20/2
  Add4/1 -> Gain/1
  Constant10/1 -> Product20/1
  Gain/1 -> Out1/1
  Constant/1 -> Product19/1
  In1/1 -> Product19/2
  Product19/1 -> Add4/1
  Product20/1 -> Add4/2

== system Simulink_Control_BlueROVtest6/Sliding Mode Control/C(v)/Subsystem22 ==
  In1 : Inport
  In2 : Inport  Port=2
  In3 : Inport  Port=3
  In4 : Inport  Port=4
  Add4 : Sum  Inputs=+++
  Add8 : Sum
  Constant : Constant  Value=-Iyz
  Constant1 : Constant  Value=Iy
  Constant10 : Constant  Value=-Ixy
  Constant11 : Constant  Value=-Mqdot
  Product{1,19..21} (4 alike) : Product
  Out1 : Outport  VectorParamsAs1DForOutWhenUnconnected=off
  wires:
  In2/1 -> Product20/2
  In1/1 -> Product19/2
  Add8/1 -> Out1/1
  Constant10/1 -> Product20/1
  Product21/1 -> Add8/2
  Constant/1 -> Product19/1
  Product19/1 -> Add4/1
  Add4/1 -> Add8/1
  Constant11/1 -> Product21/1
  Product20/1 -> Add4/2
  Product1/1 -> Add4/3
  Constant1/1 -> Product1/1
  In4/1 -> Product21/2
  In3/1 -> Product1/2

== system Simulink_Control_BlueROVtest6/Sliding Mode Control/C(v)/Subsystem23 ==
  In1 : Inport
  In2 : Inport  Port=2
  In3 : Inport  Port=3
  In4 : Inport  Port=4
  Add4 : Sum  Inputs=+++
  Add8 : Sum
  Constant : Constant  Value=Ixz
  Constant1 : Constant  Value=-Ix
  Constant10 : Constant  Value=Ixy
  Constant11 : Constant  Value=Kpdot
  Product{1,19..21} (4 alike) : Product
  Out1 : Outport  VectorParamsAs1DForOutWhenUnconnected=off
  wires:
  In3/1 -> Product1/2
  In4/1 -> Product21/2
  Constant1/1 -> Product1/1
  Product1/1 -> Add4/3
  Product20/1 -> Add4/2
  Constant11/1 -> Product21/1
  Add4/1 -> Add8/1
  Product19/1 -> Add4/1
  Constant/1 -> Product19/1
  Product21/1 -> Add8/2
  Constant10/1 -> Product20/1
  Add8/1 -> Out1/1
  In1/1 -> Product19/2
  In2/1 -> Product20/2

== system Simulink_Control_BlueROVtest6/Sliding Mode Control/C(v)/Subsystem3 ==
  In1 : Inport
  In2 : Inport  Port=2
  In3 : Inport  Port=3
  Add4 : Sum
  Add8 : Sum  Inputs=-+
  Constant : Constant  Value=yg
  Constant10 : Constant
  Constant11 : Constant  Value=Zwdot
  Gain : Gain  Gain=m
  Product19 : Product
  Product20 : Product
  Product21 : Product
  Out1 : Outport  VectorParamsAs1DForOutWhenUnconnected=off
  wires:
  In2/1 -> Product20/2
  In3/1 -> Product21/2
  In1/1 -> Product19/2
  Add8/1 -> Out1/1
  Constant10/1 -> Product20/1
  Add4/1 -> Gain/1
  Product21/1 -> Add8/2
  Constant/1 -> Product19/1
  Product19/1 -> Add4/1
  Gain/1 -> Add8/1
  Constant11/1 -> Product21/1
  Product20/1 -> Add4/2

== system Simulink_Control_BlueROVtest6/Sliding Mode Control/C(v)/Subsystem4 ==
  In1 : Inport
  In2 : Inport  Port=2
  Add4 : Sum
  Constant : Constant  Value=zg
  Constant10 : Constant  Value=xg
  Gain : Gain  Gain=m
  Product19 : Product
  Product20 : Product
  Out1 : Outport  VectorParamsAs1DForOutWhenUnconnected=off
  wires:
  In2/1 -> Product20/2
  Add4/1 -> Gain/1
  Constant10/1 -> Product20/1
  Gain/1 -> Out1/1
  Constant/1 -> Product19/1
  In1/1 -> Product19/2
  Product19/1 -> Add4/1
  Product20/1 -> Add4/2

== system Simulink_Control_BlueROVtest6/Sliding Mode Control/C(v)/Subsystem5 ==
  In1 : Inport
  In2 : Inport  Port=2
  In3 : Inport  Port=3
  Add4 : Sum  Inputs=+-
  Add8 : Sum  Inputs=-+
  Constant : Constant  Value=yg
  Constant10 : Constant
  Constant11 : Constant  Value=-Xudot
  Gain : Gain  Gain=m
  Product19 : Product
  Product20 : Product
  Product21 : Product
  Out1 : Outport  VectorParamsAs1DForOutWhenUnconnected=off
  wires:
  Product20/1 -> Add4/2
  Constant11/1 -> Product21/1
  Gain/1 -> Add8/1
  Product19/1 -> Add4/1
  Constant/1 -> Product19/1
  Product21/1 -> Add8/2
  Add4/1 -> Gain/1
  Constant10/1 -> Product20/1
  Add8/1 -> Out1/1
  In1/1 -> Product19/2
  In3/1 -> Product21/2
  In2/1 -> Product20/2

== system Simulink_Control_BlueROVtest6/Sliding Mode Control/C(v)/Subsystem6 ==
  In1 : Inport
  In2 : Inport  Port=2
  In3 : Inport  Port=3
  Add4 : Sum  Inputs=+-
  Add8 : Sum  Inputs=-+
  Constant : Constant  Value=zg
  Constant10 : Constant
  Constant11 : Constant  Value=-Yvdot
  Gain : Gain  Gain=m
  Product19 : Product
  Product20 : Product
  Product21 : Product
  Out1 : Outport  VectorParamsAs1DForOutWhenUnconnected=off
  wires:
  In2/1 -> Product20/2
  In3/1 -> Product21/2
  In1/1 -> Product19/2
  Add8/1 -> Out1/1
  Constant10/1 -> Product20/1
  Add4/1 -> Gain/1
  Product21/1 -> Add8/2
  Constant/1 -> Product19/1
  Product19/1 -> Add4/1
  Gain/1 -> Add8/1
  Constant11/1 -> Product21/1
  Product20/1 -> Add4/2

== system Simulink_Control_BlueROVtest6/Sliding Mode Control/C(v)/Subsystem7 ==
  In1 : Inport
  In2 : Inport  Port=2
  In3 : Inport  Port=3
  Add4 : Sum
  Add8 : Sum  Inputs=-+
  Constant : Constant  Value=zg
  Constant10 : Constant
  Constant11 : Constant  Value=Xudot
  Gain : Gain  Gain=m
  Product19 : Product
  Product20 : Product
  Product21 : Product
  Out1 : Outport  VectorParamsAs1DForOutWhenUnconnected=off
  wires:
  Product20/1 -> Add4/2
  Constant11/1 -> Product21/1
  Gain/1 -> Add8/1
  Product19/1 -> Add4/1
  Constant/1 -> Product19/1
  Product21/1 -> Add8/2
  Add4/1 -> Gain/1
  Constant10/1 -> Product20/1
  Add8/1 -> Out1/1
  In1/1 -> Product19/2
  In3/1 -> Product21/2
  In2/1 -> Product20/2

== system Simulink_Control_BlueROVtest6/Sliding Mode Control/C(v)/Subsystem8 ==
  In1 : Inport
  In2 : Inport  Port=2
  Add4 : Sum
  Constant : Constant  Value=xg
  Constant10 : Constant  Value=yg
  Gain : Gain  Gain=m
  Product19 : Product
  Product20 : Product
  Out1 : Outport  VectorParamsAs1DForOutWhenUnconnected=off
  wires:
  In2/1 -> Product20/2
  Add4/1 -> Gain/1
  Constant10/1 -> Product20/1
  Gain/1 -> Out1/1
  Constant/1 -> Product19/1
  In1/1 -> Product19/2
  Product19/1 -> Add4/1
  Product20/1 -> Add4/2

== system Simulink_Control_BlueROVtest6/Sliding Mode Control/C(v)/Subsystem9 ==
  In1 : Inport
  In2 : Inport  Port=2
  Add4 : Sum
  Constant : Constant  Value=yg
  Constant10 : Constant  Value=zg
  Gain : Gain  Gain=-m
  Product19 : Product
  Product20 : Product
  Out1 : Outport  VectorParamsAs1DForOutWhenUnconnected=off
  wires:
  In2/1 -> Product20/2
  Add4/1 -> Gain/1
  Constant10/1 -> Product20/1
  Gain/1 -> Out1/1
  Constant/1 -> Product19/1
  In1/1 -> Product19/2
  Product19/1 -> Add4/1
  Product20/1 -> Add4/2
